simulink model "AMM_tracking"  (R2020a)
settings: Solver=VariableStepAuto  StartTime=0.0  StopTime=350  RelTol=1e-3
values from neighbouring files (symbols this model uses):
  a = (6371+h)*1e3    (= 6871000)    [AMM_main.m]    (also in Data.m)
  A_RW = sqrt([prop1;prop2;prop3]/(prop1+prop2+prop3))    [AMM_main.m]    (also in Data.m)
  A_t = [Ax;Ay;Az;Ax;Ay;Az;A_sp;A_sp;A_sp;A_sp;]    [AMM_main.m]    (also in Data.m)
  alpha = 0.005    [AMM_main.m]    (also in Data.m = 0.5)
  cd = 2.2    [AMM_main.m]    (also in Data.m)
  EH_dir = [0.152451072968615, 0.104990641908259, -0.112754568516865]    [AMM_main.m]
  EH_err = 0.25*pi/180    (= 0.00436332312999)    [AMM_main.m]
  Gyr_frq = 262    [AMM_main.m]
  init_DCM = DCM0_track    [AMM_main.m]    (also in Data.m = [0.097540404999410   0.957506835434298   0.970592781760616)
  init_gyro = w0_gyro_track    [AMM_main.m]
  init_hr = hr0_track    [AMM_main.m]
  init_orb = orb0_track    [AMM_main.m]    (also in Data.m = [e0,i0,O0,o0,th0])
  init_tumbl = w0_track    [AMM_main.m]    (also in Data.m = 10*pi/180*dir)
  Ir = 1e-7    (= 1e-07)    [AMM_main.m]    (also in Data.m)
  J = [Jx;Jy;Jz]    [AMM_main.m]    (also in Data.m)
  K1 = .05    (= 0.05)    [AMM_main.m]    (also in Data.m)
  K2 = 0.5*K1^2    (= 0.00125)    [AMM_main.m]    (also in Data.m)
  max_mx = 1.19    [AMM_main.m]    (also in Data.m)
  max_my = 1.19    [AMM_main.m]    (also in Data.m)
  MS_dir = [-0.144926348121151, 0.497003271606648, -0.275828501016873]    [AMM_main.m]
  MS_err = 2*pi/180    (= 0.0349065850399)    [AMM_main.m]
  MS_freq = 1    [AMM_main.m]    (also in Data.m)
  n = sqrt( mu / a^3 )    [AMM_main.m]    (also in Data.m)
  par_ind = [0.1;0.1;0.1]    [AMM_main.m]
  rho = [rho_sMB;rho_dMB;rho_sSP;rho_dSP]    [AMM_main.m]    (also in Data.m)
  rho_air = 4.39e-16 * 1e6/1e3    (= 4.39e-13)    [AMM_main.m]    (also in Data.m)
  RW_max_momentum = 400e-3    (= 0.4)    [AMM_main.m]    (also in Data.m)
  RW_max_torque = 100e-3    (= 0.1)    [AMM_main.m]    (also in Data.m)
  t0 = de_tumble.tout(end)    [AMM_main.m]
  wr = 100*pi/180    (= 1.74532925199)    [AMM_main.m]    (also in Data.m)
  ww_earth = 2*pi/(24*3600)*[0;0;1]    [AMM_main.m]    (also in Data.m)
libraries: dspmtrx3 x3, vrlib x3, simulink x3
(part 1 of 2)
settings Model: Creator=alejandrodemiguelmendiola  LastModifiedBy=alejandrodemiguelmendiola

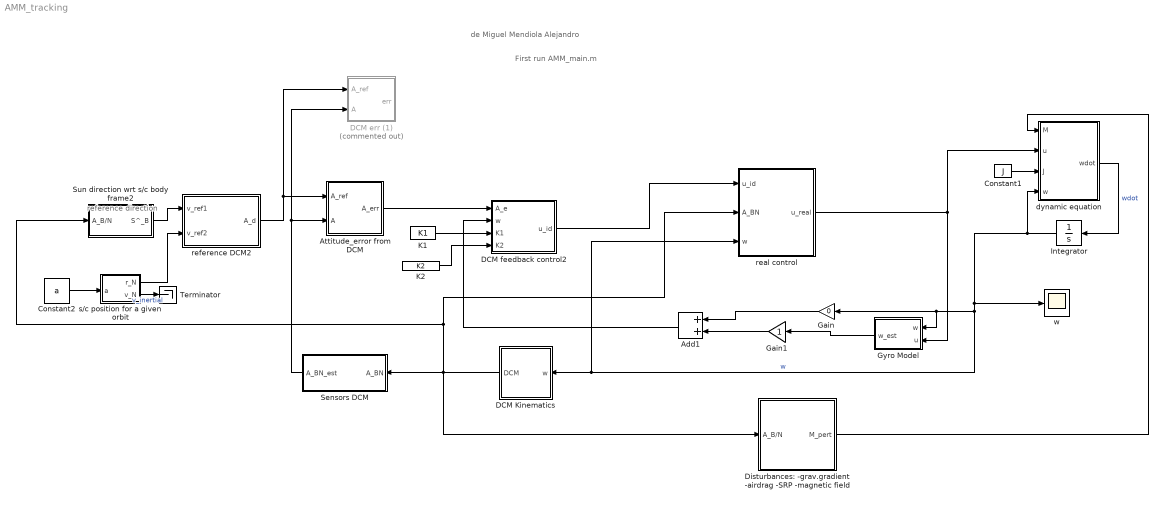
== system AMM_tracking ==
  note: reference direction
  note: First run AMM_main.m
  note: de Miguel Mendiola Alejandro
  Add1 : Sum
  Attitude_error from DCM : Subsystem
  Constant1 : Constant  Value=J
  Constant2 : Constant  Value=a
  DCM Kinematics : Subsystem
  DCM err (1) : Subsystem  Commented=on
  DCM feedback control2 : Subsystem
  Disturbances: -grav.gradient -airdrag -SRP -magnetic field : Subsystem
  Gain : Gain  Gain=0
  Gain1 : Gain
  Gyro Model : Subsystem
  Integrator : Integrator  InitialCondition=init_tumbl
  K1 : Constant  Value=K1
  K2 : Constant  Value=K2
  Sensors DCM : Subsystem
  Sun direction wrt s/c body frame2 : Subsystem
  Terminator : Terminator
  dynamic equation : MATLAB Function  TreatAsAtomicUnit=on
  "real control " : Subsystem
  reference DCM2 : Subsystem
  s/c position for a given orbit : Subsystem
  w : Scope
  wires:
  dynamic equation/1(wdot) -> Integrator/1  "wdot"
  Integrator/1 -> w/1, "real control "/3(w), DCM Kinematics/1(w), Gyro Model/1(w), Gain/1, dynamic equation/4(w)  "w"
  Disturbances: -grav.gradient -airdrag -SRP -magnetic field/1(M_pert) -> dynamic equation/1(M)
  Constant1/1 -> dynamic equation/3(J)
  Add1/1 -> DCM feedback control2/2(w)
  Gain1/1 -> Add1/2
  Gyro Model/1(w_est) -> Gain1/1
  Gain/1 -> Add1/1
  reference DCM2/1(A_d) -> DCM err (1)/1(A_ref), Attitude_error from DCM/1(A_ref)
  DCM Kinematics/1(DCM) -> "real control "/2(A_BN), Sun direction wrt s/c body frame2/1(A_B/N), Disturbances: -grav.gradient -airdrag -SRP -magnetic field/1(A_B/N), Sensors DCM/1(A_BN)
  Attitude_error from DCM/1(A_err) -> DCM feedback control2/1(A_e)
  Sensors DCM/1(A_BN_est) -> DCM err (1)/2(A), Attitude_error from DCM/2(A)
  K1/1 -> DCM feedback control2/3(K1)
  K2/1 -> DCM feedback control2/4(K2)
  Constant2/1 -> s/c position for a given orbit/1(a)
  s/c position for a given orbit/2(v_N) -> Terminator/1  "v_inertial"
  s/c position for a given orbit/1(r_N) -> reference DCM2/2(v_ref2)
  Sun direction wrt s/c body frame2/1(S^_B) -> reference DCM2/1(v_ref1)
  "real control "/1(u_real) -> dynamic equation/2(u), Gyro Model/2(u)
  DCM feedback control2/1(u_id) -> "real control "/1(u_id)

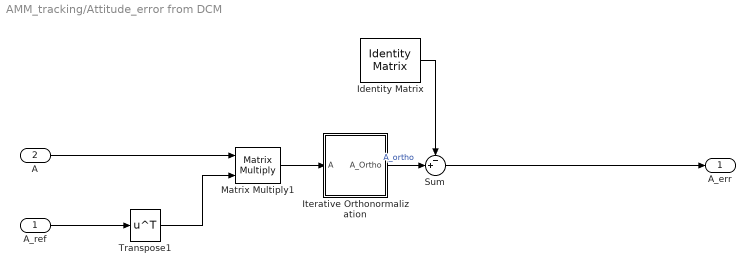
== system AMM_tracking/Attitude_error from DCM ==
  A_ref : Inport
  A : Inport  Port=2
  Identity Matrix : dspmtrx3/Identity Matrix  Inherit=off  N=3  Ts=1  dataType=double  isSigned=on  wordLen=16  udDataType=sfix(16)  fracBitsMode=Best precision  numFracBits=15  OutDataTypeStr=double  LastOutDataTypeStr=double
  Iterative Orthonormalization : Subsystem
  Matrix Multiply1 : Product  Multiplication=Matrix(*)
  Sum : Sum  Inputs=-+|
  Transpose1 : Math  Operator=transpose  SaturateOnIntegerOverflow=on
  A_err : Outport
  wires:
  A_ref/1 -> Transpose1/1
  Transpose1/1 -> Matrix Multiply1/2
  A/1 -> Matrix Multiply1/1
  Sum/1 -> A_err/1
  Identity Matrix/1 -> Sum/1
  Matrix Multiply1/1 -> Iterative Orthonormalization/1(A)
  Iterative Orthonormalization/1(A_Ortho) -> Sum/2  "A_ortho"

== system AMM_tracking/DCM Kinematics ==
  w : Inport
  Integrator : Integrator  InitialCondition=init_DCM
  Iterative Orthonormalization : Subsystem
  Product1 : Product  Multiplication=Matrix(*)
  Unary Minus : UnaryMinus
  hat : MATLAB Function  TreatAsAtomicUnit=on
  DCM : Outport
  wires:
  Unary Minus/1 -> Integrator/1  "Adot"
  hat/1(w_hat) -> Product1/1
  Product1/1 -> Unary Minus/1
  w/1 -> hat/1(w)
  Iterative Orthonormalization/1(A_Ortho) -> Product1/2, DCM/1  "A_ortho"
  Integrator/1 -> Iterative Orthonormalization/1(A)  "A"

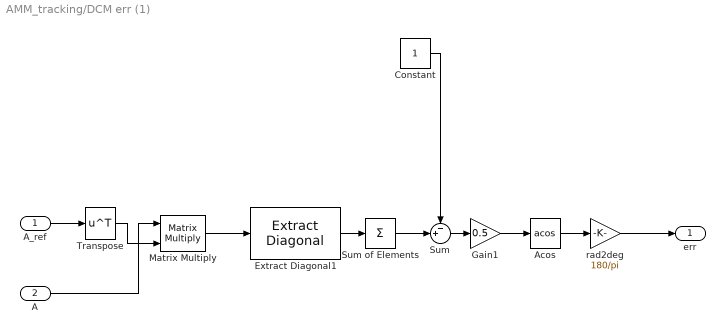
== system AMM_tracking/DCM err (1) ==
  A_ref : Inport
  A : Inport  Port=2
  Acos : Trigonometry  Operator=acos
  Constant : Constant
  Extract Diagonal1 : dspmtrx3/Extract Diagonal
      settings: SourceProductBaseCode=DS
  Gain1 : Gain  Gain=0.5
  Matrix Multiply : Product  Multiplication=Matrix(*)
  Sum : Sum  Inputs=-+|
  Sum of Elements : Sum  Inputs=+
  Transpose : Math  Operator=transpose  SaturateOnIntegerOverflow=on
  rad2deg : Gain  Gain=180/pi
  err : Outport
  wires:
  Matrix Multiply/1 -> Extract Diagonal1/1
  Extract Diagonal1/1 -> Sum of Elements/1
  A_ref/1 -> Transpose/1
  Sum/1 -> Gain1/1
  Acos/1 -> rad2deg/1
  Sum of Elements/1 -> Sum/2
  Constant/1 -> Sum/1
  rad2deg/1 -> err/1
  Gain1/1 -> Acos/1
  A/1 -> Matrix Multiply/1
  Transpose/1 -> Matrix Multiply/2

== system AMM_tracking/DCM feedback control2 ==
  A_e : Inport
  w : Inport  Port=2
  K1 : Inport  Port=3
  K2 : Inport  Port=4
  Constant2 : Constant  Value=J
  DCM feedback : MATLAB Function  TreatAsAtomicUnit=on
  u_id : Outport
  wires:
  DCM feedback/1(u) -> u_id/1
  A_e/1 -> DCM feedback/2(A_e)
  Constant2/1 -> DCM feedback/5(J)
  K2/1 -> DCM feedback/4(K2)
  w/1 -> DCM feedback/1(w)
  K1/1 -> DCM feedback/3(K1)

== system AMM_tracking/Disturbances: -grav.gradient -airdrag -SRP -magnetic field ==
  A_B/N : Inport
  Add : Sum  Inputs=++++
  SRP moment : Subsystem
  air drag : Subsystem
  gravity gradient : Subsystem
  magnetic torque : Subsystem
  M_pert : Outport
  wires:
  magnetic torque/1(magnetic torque M) -> Add/1
  SRP moment/1(T_srp) -> Add/2
  gravity gradient/1(G) -> Add/4
  Add/1 -> M_pert/1
  air drag/1(M_drag) -> Add/3
  A_B/N/1 -> magnetic torque/1(A_BN), SRP moment/1(A_B/N), gravity gradient/1(A_BN), air drag/1(A_B/N)

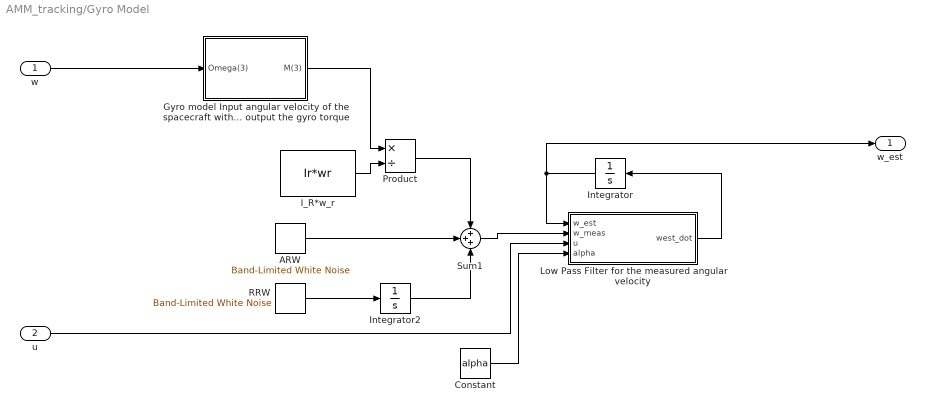
== system AMM_tracking/Gyro Model ==
  w : Inport
  u : Inport  Port=2
  ARW : simulink/Sources/Band-Limited White Noise  Cov=Gyr_ARW  Ts=1/Gyr_frq  seed=[23341]
  Constant : Constant  Value=alpha
  Gyro model Input angular velocity of the spacecraft with output the gyro torque : Subsystem
  I_R*w_r : Constant  Value=Ir*wr
  Integrator : Integrator  InitialCondition=init_gyro
  Integrator2 : Integrator  InitialCondition=pi/180/3600*[1,1,1]'
  Low Pass Filter for the measured angular velocity : MATLAB Function  TreatAsAtomicUnit=on
  Product : Product  Inputs=*/
  RRW : simulink/Sources/Band-Limited White Noise  Cov=Gyr_RRW  Ts=1/Gyr_frq  seed=[23341]
  Sum1 : Sum  Inputs=+++
  w_est : Outport
  wires:
  Gyro model Input angular velocity of the spacecraft with output the gyro torque/1(M(3)) -> Product/1
  Low Pass Filter for the measured angular velocity/1(west_dot) -> Integrator/1
  I_R*w_r/1 -> Product/2
  Integrator/1 -> w_est/1, Low Pass Filter for the measured angular velocity/1(w_est)
  Sum1/1 -> Low Pass Filter for the measured angular velocity/2(w_meas)
  w/1 -> Gyro model Input angular velocity of the spacecraft with output the gyro torque/1(Omega(3))
  u/1 -> Low Pass Filter for the measured angular velocity/3(u)
  Integrator2/1 -> Sum1/3
  Product/1 -> Sum1/1
  RRW/1 -> Integrator2/1
  ARW/1 -> Sum1/2
  Constant/1 -> Low Pass Filter for the measured angular velocity/4(alpha)

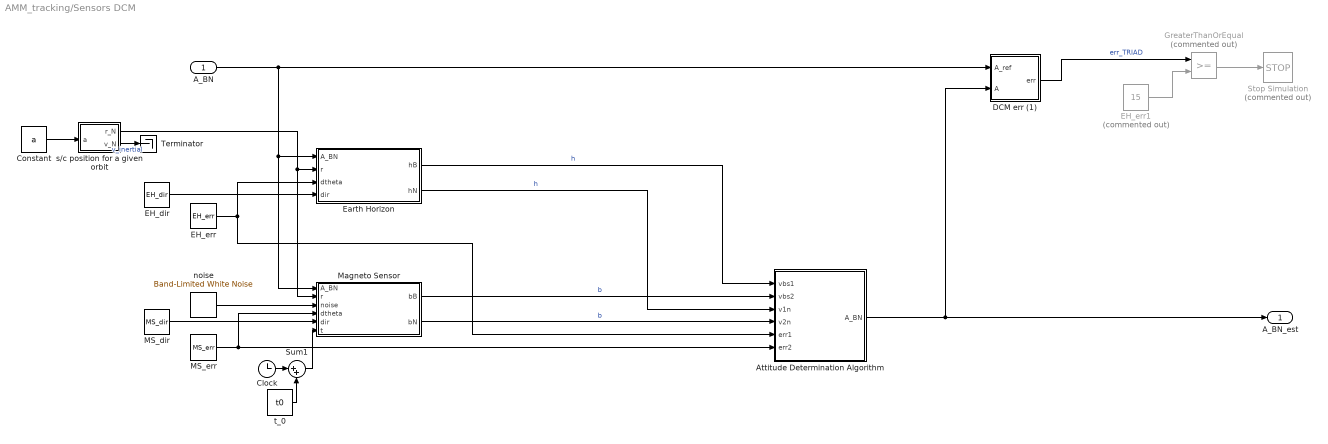
== system AMM_tracking/Sensors DCM ==
  A_BN : Inport
  Attitude Determination Algorithm : MATLAB Function  TreatAsAtomicUnit=on
  Clock : Clock
  Constant : Constant  Value=a
  DCM err (1) : Subsystem
  EH_dir : Constant  Value=EH_dir
  EH_err : Constant  Value=EH_err
  EH_err1 : Constant  Commented=on  Value=15
  Earth Horizon : MATLAB Function  TreatAsAtomicUnit=on
  GreaterThanOrEqual : RelationalOperator  Commented=on  OutDataTypeStr=boolean  RndMeth=Simplest
  MS_dir : Constant  Value=MS_dir
  MS_err : Constant  Value=MS_err
  Magneto Sensor : MATLAB Function  TreatAsAtomicUnit=on
  Stop Simulation : Stop  Commented=on
  Sum1 : Sum  Inputs=|++
  Terminator : Terminator
  noise : simulink/Sources/Band-Limited White Noise  Cov=MS_noise  Ts=MS_freq  seed=[23341]
  s/c position for a given orbit : Subsystem
  t_0 : Constant  Value=t0
  A_BN_est : Outport
  wires:
  s/c position for a given orbit/1(r_N) -> Earth Horizon/2(r), Magneto Sensor/2(r)
  EH_err/1 -> Earth Horizon/3(dtheta), Attitude Determination Algorithm/5(err1)
  Earth Horizon/1(hB) -> Attitude Determination Algorithm/1(vbs1)  "h"
  MS_err/1 -> Magneto Sensor/4(dtheta), Attitude Determination Algorithm/6(err2)
  Magneto Sensor/1(bB) -> Attitude Determination Algorithm/2(vbs2)  "b"
  Clock/1 -> Sum1/1
  A_BN/1 -> DCM err (1)/1(A_ref), Magneto Sensor/1(A_BN), Earth Horizon/1(A_BN)
  DCM err (1)/1(err) -> GreaterThanOrEqual/1  "err_TRIAD"
  Attitude Determination Algorithm/1(A_BN) -> A_BN_est/1, DCM err (1)/2(A)
  Sum1/1 -> Magneto Sensor/6(t)
  noise/1 -> Magneto Sensor/3(noise)
  MS_dir/1 -> Magneto Sensor/5(dir)
  EH_dir/1 -> Earth Horizon/4(dir)
  t_0/1 -> Sum1/2
  Earth Horizon/2(hN) -> Attitude Determination Algorithm/3(v1n)  "h"
  Magneto Sensor/2(bN) -> Attitude Determination Algorithm/4(v2n)  "b"
  GreaterThanOrEqual/1 -> Stop Simulation/1
  EH_err1/1 -> GreaterThanOrEqual/2
  Constant/1 -> s/c position for a given orbit/1(a)
  s/c position for a given orbit/2(v_N) -> Terminator/1  "v_inertial"

== system AMM_tracking/Sun direction wrt s//c body frame2 ==
  A_B/N : Inport
  Add : Sum
  Clock : Clock
  Constant1 : Constant  Value=t0
  Product3 : Product  Multiplication=Matrix(*)
  Sun's direction : MATLAB Function  TreatAsAtomicUnit=on
  S^_B : Outport
  wires:
  Product3/1 -> S^_B/1
  A_B/N/1 -> Product3/1
  Sun's direction/1(S_N) -> Product3/2  "S^_N"
  Clock/1 -> Add/1
  Add/1 -> Sun's direction/1(t)
  Constant1/1 -> Add/2

== system AMM_tracking/real control  ==
  u_id : Inport
  A_BN : Inport  Port=2
  w : Inport  Port=3
  Add : Sum
  MT+RW control1 : Subsystem  Commented=on
  RW : Subsystem
  u_real : Outport
  wires:
  RW/1(u_r) -> Add/1  "u_real 4RW"
  w/1 -> RW/2(w), MT+RW control1/1(w)
  A_BN/1 -> MT+RW control1/3(A_BN)
  Add/1 -> u_real/1
  MT+RW control1/1(u_real) -> Add/2
  u_id/1 -> RW/1(u_id), MT+RW control1/2(M_c)

== system AMM_tracking/reference DCM2 ==
  v_ref1 : Inport
  v_ref2 : Inport  Port=2
  DCM_ref : MATLAB Function  TreatAsAtomicUnit=on
  A_d : Outport
  wires:
  DCM_ref/1(A_d) -> A_d/1
  v_ref1/1 -> DCM_ref/1(v_ref)
  v_ref2/1 -> DCM_ref/2(r_sc)

== system AMM_tracking/s//c position for a given orbit ==
  a : Inport
  Earth's position : MATLAB Function  TreatAsAtomicUnit=on
  orb_elements dynamics : Subsystem
  r_N : Outport
  v_N : Outport  Port=2
  wires:
  Earth's position/1(r_N) -> r_N/1  "r_N"
  orb_elements dynamics/1(orb_elements) -> Earth's position/2(orb_elements)
  a/1 -> orb_elements dynamics/1(a), Earth's position/1(a)  "a"
  Earth's position/2(v_N) -> v_N/1

== system AMM_tracking/Attitude_error from DCM/Iterative Orthonormalization ==
  note: Uncomment if needed
      | With 2 blocks working:
      | Error ~1e-16 up to t=1e6
      | Error ~1e-14 up to t=1e7
  A : Inport
  Ortho DCM : Subsystem
  Ortho DCM1 : Subsystem
  Ortho DCM2 : Subsystem
  Ortho DCM3 : Subsystem  Commented=through
  Ortho DCM4 : Subsystem  Commented=through
  A_Ortho : Outport
  wires:
  Ortho DCM1/1(A_ortho) -> Ortho DCM2/1(A)
  Ortho DCM/1(A_ortho) -> Ortho DCM1/1(A)
  Ortho DCM3/1(A_ortho) -> Ortho DCM4/1(A)
  Ortho DCM2/1(A_ortho) -> Ortho DCM3/1(A)
  A/1 -> Ortho DCM/1(A)
  Ortho DCM4/1(A_ortho) -> A_Ortho/1

== system AMM_tracking/DCM Kinematics/Iterative Orthonormalization ==
  note: Uncomment if needed
      | With 2 blocks working:
      | Error ~1e-16 up to t=1e6
      | Error ~1e-14 up to t=1e7
  A : Inport
  Ortho DCM : Subsystem
  Ortho DCM1 : Subsystem
  Ortho DCM2 : Subsystem  Commented=through
  Ortho DCM3 : Subsystem  Commented=through
  Ortho DCM4 : Subsystem  Commented=through
  A_Ortho : Outport
  wires:
  Ortho DCM1/1(A_ortho) -> Ortho DCM2/1(A)
  Ortho DCM/1(A_ortho) -> Ortho DCM1/1(A)
  Ortho DCM3/1(A_ortho) -> Ortho DCM4/1(A)
  Ortho DCM2/1(A_ortho) -> Ortho DCM3/1(A)
  A/1 -> Ortho DCM/1(A)
  Ortho DCM4/1(A_ortho) -> A_Ortho/1

== system AMM_tracking/Disturbances: -grav.gradient -airdrag -SRP -magnetic field/SRP moment ==
  A_B/N : Inport
  Area : Constant  Value=A_t
  SRP disturbance torque : MATLAB Function  TreatAsAtomicUnit=on
  Sun direction wrt s/c body frame : Subsystem
  optical properties : Constant  Value=rho
  T_srp : Outport
  wires:
  A_B/N/1 -> Sun direction wrt s/c body frame/1(A_B/N)
  SRP disturbance torque/1(T_srp) -> T_srp/1
  Sun direction wrt s/c body frame/1(S^_B) -> SRP disturbance torque/1(S_B)
  Area/1 -> SRP disturbance torque/2(A)
  optical properties/1 -> SRP disturbance torque/3(rho)

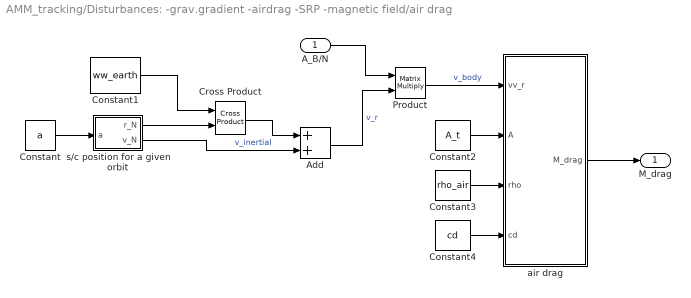
== system AMM_tracking/Disturbances: -grav.gradient -airdrag -SRP -magnetic field/air drag ==
  A_B/N : Inport
  Add : Sum
  Constant : Constant  Value=a
  Constant1 : Constant  Value=ww_earth
  Constant2 : Constant  Value=A_t
  Constant3 : Constant  Value=rho_air
  Constant4 : Constant  Value=cd
  Cross Product : vrlib/Utilities/Cross Product
  Product : Product  Multiplication=Matrix(*)
  air drag : MATLAB Function  TreatAsAtomicUnit=on
  s/c position for a given orbit : Subsystem
  M_drag : Outport
  wires:
  air drag/1(M_drag) -> M_drag/1
  A_B/N/1 -> Product/1
  Product/1 -> air drag/1(vv_r)  "v_body"
  Constant/1 -> s/c position for a given orbit/1(a)
  s/c position for a given orbit/1(r_N) -> Cross Product/2
  Constant1/1 -> Cross Product/1
  Cross Product/1 -> Add/1
  s/c position for a given orbit/2(v_N) -> Add/2  "v_inertial"
  Add/1 -> Product/2  "v_r"
  Constant2/1 -> air drag/2(A)
  Constant4/1 -> air drag/4(cd)
  Constant3/1 -> air drag/3(rho)

== system AMM_tracking/Disturbances: -grav.gradient -airdrag -SRP -magnetic field/gravity gradient ==
  A_BN : Inport
  A_N/L : Subsystem
  Product : Product  Multiplication=Matrix(*)
  gravity gradient : MATLAB Function  TreatAsAtomicUnit=on
  mean motion : Constant  Value=n
  moment of inertia : Constant  Value=J
  G : Outport
  wires:
  gravity gradient/1(G) -> G/1
  A_N/L/1(A_N/L) -> Product/2
  A_BN/1 -> Product/1
  Product/1 -> gravity gradient/1(A_BL)
  moment of inertia/1 -> gravity gradient/2(J)
  mean motion/1 -> gravity gradient/3(n)

== system AMM_tracking/Disturbances: -grav.gradient -airdrag -SRP -magnetic field/magnetic torque ==
  A_BN : Inport
  Cross Product : vrlib/Utilities/Cross Product
  m (worst case scenario) : Constant  Value=par_ind
  magnetic model : Subsystem
  magnetic torque M : Outport
  wires:
  magnetic model/1(b_B) -> Cross Product/2  "b_B"
  m (worst case scenario)/1 -> Cross Product/1
  Cross Product/1 -> magnetic torque M/1  "M"
  A_BN/1 -> magnetic model/1(A_BN)

== system AMM_tracking/Gyro Model/Gyro model Input angular velocity of the spacecraft with output the gyro torque ==
  Omega(3) : Inport
  Integrator2 : Integrator  InitialCondition=[0;0;0;0;0;0]
  MATLAB Function1 : MATLAB Function  TreatAsAtomicUnit=on
  M(3) : Outport
  wires:
  Integrator2/1 -> MATLAB Function1/1(x)
  MATLAB Function1/1(x_dot) -> Integrator2/1
  Omega(3)/1 -> MATLAB Function1/2(om)
  MATLAB Function1/2(M) -> M(3)/1

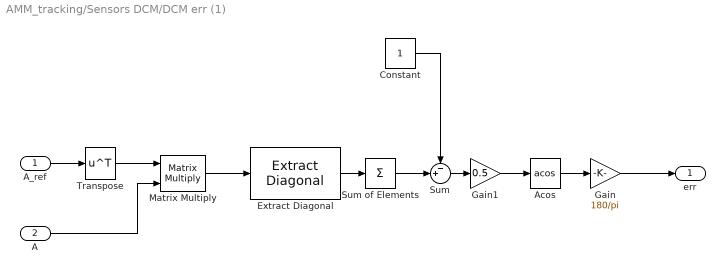
== system AMM_tracking/Sensors DCM/DCM err (1) ==
  A_ref : Inport
  A : Inport  Port=2
  Acos : Trigonometry  Operator=acos
  Constant : Constant
  Extract Diagonal : dspmtrx3/Extract Diagonal
      settings: SourceProductBaseCode=DS
  Gain : Gain  Gain=180/pi
  Gain1 : Gain  Gain=0.5
  Matrix Multiply : Product  Multiplication=Matrix(*)
  Sum : Sum  Inputs=-+|
  Sum of Elements : Sum  Inputs=+
  Transpose : Math  Operator=transpose  SaturateOnIntegerOverflow=on
  err : Outport
  wires:
  Transpose/1 -> Matrix Multiply/1
  Matrix Multiply/1 -> Extract Diagonal/1
  Extract Diagonal/1 -> Sum of Elements/1
  A/1 -> Matrix Multiply/2
  A_ref/1 -> Transpose/1
  Sum/1 -> Gain1/1
  Acos/1 -> Gain/1
  Sum of Elements/1 -> Sum/2
  Constant/1 -> Sum/1
  Gain/1 -> err/1
  Gain1/1 -> Acos/1

== system AMM_tracking/Sensors DCM/s//c position for a given orbit ==
  a : Inport
  Earth's position : MATLAB Function  TreatAsAtomicUnit=on
  orb_elements dynamics : Subsystem
  r_N : Outport
  v_N : Outport  Port=2
  wires:
  Earth's position/1(r_N) -> r_N/1  "r_N"
  orb_elements dynamics/1(orb_elements) -> Earth's position/2(orb_elements)
  a/1 -> orb_elements dynamics/1(a), Earth's position/1(a)  "a"
  Earth's position/2(v_N) -> v_N/1

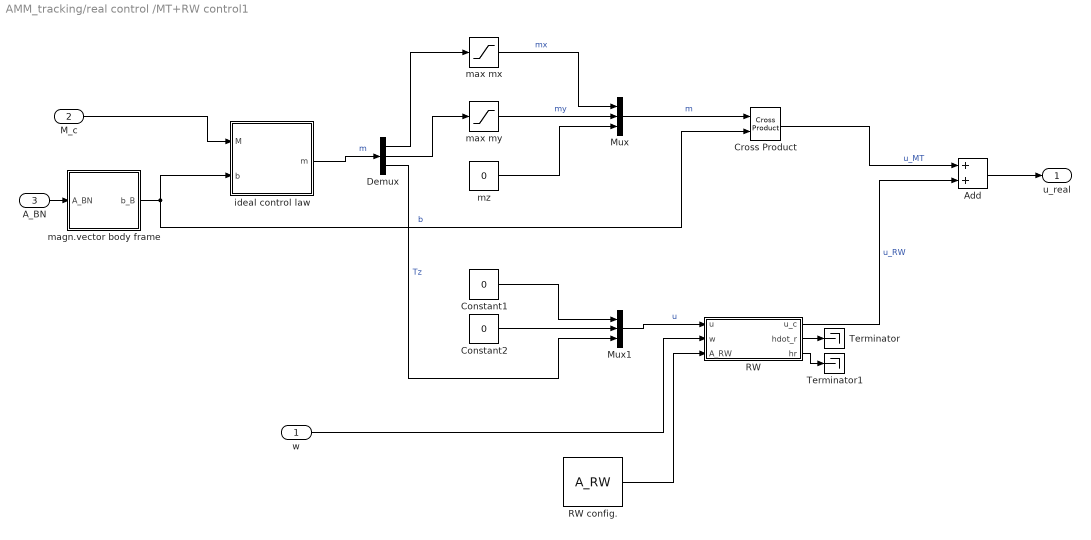
== system AMM_tracking/real control /MT+RW control1 ==
  w : Inport
  M_c : Inport  Port=2
  A_BN : Inport  Port=3
  " RW" : Subsystem
  Add : Sum
  Constant1 : Constant  Value=0
  Constant2 : Constant  Value=0
  Cross Product : vrlib/Utilities/Cross Product
  Demux : Demux  Outputs=3
  Mux : Mux  Inputs=3
  Mux1 : Mux  Inputs=3
  RW config. : Constant  Value=A_RW
  Terminator : Terminator
  Terminator1 : Terminator
  ideal control law : MATLAB Function  TreatAsAtomicUnit=on
  magn.vector body frame : Subsystem
  max mx : Saturate  UpperLimit=max_mx  LowerLimit=-max_mx
  max my : Saturate  UpperLimit=max_my  LowerLimit=-max_my
  mz : Constant  Value=0
  u_real : Outport
  wires:
  magn.vector body frame/1(b_B) -> Cross Product/2, ideal control law/2(b)  "b"
  M_c/1 -> ideal control law/1(M)
  A_BN/1 -> magn.vector body frame/1(A_BN)
  ideal control law/1(m) -> Demux/1  "m"
  Mux/1 -> Cross Product/1  "m"
  max mx/1 -> Mux/1  "mx"
  Demux/2 -> max my/1
  Demux/1 -> max mx/1
  max my/1 -> Mux/2  "my"
  mz/1 -> Mux/3
  Constant2/1 -> Mux1/2
  Demux/3 -> Mux1/3  "Tz"
  Constant1/1 -> Mux1/1
  Mux1/1 -> " RW"/1(u)  "u"
  Cross Product/1 -> Add/1  "u_MT"
  w/1 -> " RW"/2(w)
  RW config./1 -> " RW"/3(A_RW)
  " RW"/1(u_c) -> Add/2  "u_RW"
  Add/1 -> u_real/1
  " RW"/2(hdot_r) -> Terminator/1
  " RW"/3(hr) -> Terminator1/1

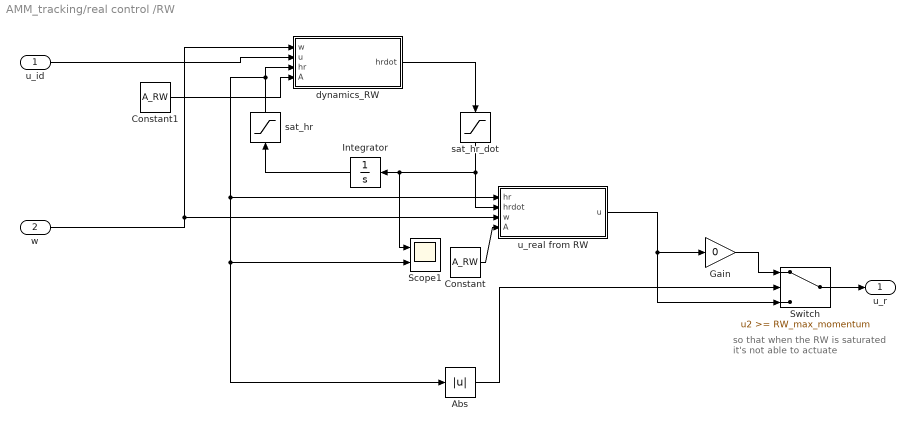
== system AMM_tracking/real control /RW ==
  note: so that when the RW is saturated
      | it's not able to actuate
  u_id : Inport
  w : Inport  Port=2
  Abs : Abs
  Constant : Constant  Value=A_RW
  Constant1 : Constant  Value=A_RW
  Gain : Gain  Gain=0
  Integrator : Integrator  InitialCondition=init_hr
  Scope1 : Scope  NumInputPorts=2
  Switch : Switch  Threshold=RW_max_momentum
  dynamics_RW : MATLAB Function  TreatAsAtomicUnit=on
  sat_hr : Saturate  UpperLimit=RW_max_momentum  LowerLimit=-RW_max_momentum
  sat_hr_dot : Saturate  UpperLimit=RW_max_torque  LowerLimit=-RW_max_torque
  u_real from RW : MATLAB Function  TreatAsAtomicUnit=on
  u_r : Outport
  wires:
  w/1 -> dynamics_RW/1(w), u_real from RW/3(w)
  u_id/1 -> dynamics_RW/2(u)
  dynamics_RW/1(hrdot) -> sat_hr_dot/1
  Integrator/1 -> sat_hr/1
  sat_hr/1 -> dynamics_RW/3(hr), Abs/1, Scope1/2, u_real from RW/1(hr)
  sat_hr_dot/1 -> Scope1/1, Integrator/1, u_real from RW/2(hrdot)
  Constant/1 -> u_real from RW/4(A)
  Constant1/1 -> dynamics_RW/4(A)
  Switch/1 -> u_r/1
  Abs/1 -> Switch/2
  u_real from RW/1(u) -> Gain/1, Switch/3
  Gain/1 -> Switch/1

== system AMM_tracking/s//c position for a given orbit/orb_elements dynamics ==
  a : Inport
  Integrator : Integrator  InitialCondition=init_orb
  sat motion : MATLAB Function  TreatAsAtomicUnit=on
  orb_elements : Outport
  wires:
  Integrator/1 -> sat motion/2(orb_elements), orb_elements/1  "orb_elements"
  sat motion/1(orb_elements_dot) -> Integrator/1
  a/1 -> sat motion/1(a)

== system AMM_tracking/Attitude_error from DCM/Iterative Orthonormalization/Ortho DCM ==
  A : Inport
  Gain : Gain  Gain=1.5
  Gain1 : Gain  Gain=0.5
  Matrix Multiply : Product  Multiplication=Matrix(*)
  Matrix Multiply1 : Product  Multiplication=Matrix(*)
  Sum : Sum  Inputs=|+-
  Transpose : Math  Operator=transpose  SaturateOnIntegerOverflow=on
  A_ortho : Outport
  wires:
  Sum/1 -> A_ortho/1
  Gain/1 -> Sum/1
  A/1 -> Matrix Multiply1/2, Transpose/1, Matrix Multiply/1, Gain/1
  Gain1/1 -> Sum/2
  Transpose/1 -> Matrix Multiply/2
  Matrix Multiply/1 -> Matrix Multiply1/1
  Matrix Multiply1/1 -> Gain1/1

== system AMM_tracking/Attitude_error from DCM/Iterative Orthonormalization/Ortho DCM1 ==
  A : Inport
  Gain : Gain  Gain=1.5
  Gain1 : Gain  Gain=0.5
  Matrix Multiply : Product  Multiplication=Matrix(*)
  Matrix Multiply1 : Product  Multiplication=Matrix(*)
  Sum : Sum  Inputs=|+-
  Transpose : Math  Operator=transpose  SaturateOnIntegerOverflow=on
  A_ortho : Outport
  wires:
  Sum/1 -> A_ortho/1
  Gain/1 -> Sum/1
  A/1 -> Matrix Multiply1/2, Transpose/1, Matrix Multiply/1, Gain/1
  Gain1/1 -> Sum/2
  Transpose/1 -> Matrix Multiply/2
  Matrix Multiply/1 -> Matrix Multiply1/1
  Matrix Multiply1/1 -> Gain1/1

== system AMM_tracking/Attitude_error from DCM/Iterative Orthonormalization/Ortho DCM2 ==
  A : Inport
  Gain : Gain  Gain=1.5
  Gain1 : Gain  Gain=0.5
  Matrix Multiply : Product  Multiplication=Matrix(*)
  Matrix Multiply1 : Product  Multiplication=Matrix(*)
  Sum : Sum  Inputs=|+-
  Transpose : Math  Operator=transpose  SaturateOnIntegerOverflow=on
  A_ortho : Outport
  wires:
  Sum/1 -> A_ortho/1
  Gain/1 -> Sum/1
  A/1 -> Matrix Multiply1/2, Transpose/1, Matrix Multiply/1, Gain/1
  Gain1/1 -> Sum/2
  Transpose/1 -> Matrix Multiply/2
  Matrix Multiply/1 -> Matrix Multiply1/1
  Matrix Multiply1/1 -> Gain1/1

== system AMM_tracking/Attitude_error from DCM/Iterative Orthonormalization/Ortho DCM3 ==
  A : Inport
  Gain : Gain  Gain=1.5
  Gain1 : Gain  Gain=0.5
  Matrix Multiply : Product  Multiplication=Matrix(*)
  Matrix Multiply1 : Product  Multiplication=Matrix(*)
  Sum : Sum  Inputs=|+-
  Transpose : Math  Operator=transpose  SaturateOnIntegerOverflow=on
  A_ortho : Outport
  wires:
  Sum/1 -> A_ortho/1
  Gain/1 -> Sum/1
  A/1 -> Matrix Multiply1/2, Transpose/1, Matrix Multiply/1, Gain/1
  Gain1/1 -> Sum/2
  Transpose/1 -> Matrix Multiply/2
  Matrix Multiply/1 -> Matrix Multiply1/1
  Matrix Multiply1/1 -> Gain1/1

== system AMM_tracking/Attitude_error from DCM/Iterative Orthonormalization/Ortho DCM4 ==
  A : Inport
  Gain : Gain  Gain=1.5
  Gain1 : Gain  Gain=0.5
  Matrix Multiply : Product  Multiplication=Matrix(*)
  Matrix Multiply1 : Product  Multiplication=Matrix(*)
  Sum : Sum  Inputs=|+-
  Transpose : Math  Operator=transpose  SaturateOnIntegerOverflow=on
  A_ortho : Outport
  wires:
  Sum/1 -> A_ortho/1
  Gain/1 -> Sum/1
  A/1 -> Matrix Multiply1/2, Transpose/1, Matrix Multiply/1, Gain/1
  Gain1/1 -> Sum/2
  Transpose/1 -> Matrix Multiply/2
  Matrix Multiply/1 -> Matrix Multiply1/1
  Matrix Multiply1/1 -> Gain1/1

== system AMM_tracking/DCM Kinematics/Iterative Orthonormalization/Ortho DCM ==
  A : Inport
  Gain : Gain  Gain=1.5
  Gain1 : Gain  Gain=0.5
  Matrix Multiply : Product  Multiplication=Matrix(*)
  Matrix Multiply1 : Product  Multiplication=Matrix(*)
  Sum : Sum  Inputs=|+-
  Transpose : Math  Operator=transpose  SaturateOnIntegerOverflow=on
  A_ortho : Outport
  wires:
  Sum/1 -> A_ortho/1
  Gain/1 -> Sum/1
  A/1 -> Matrix Multiply1/2, Transpose/1, Matrix Multiply/1, Gain/1
  Gain1/1 -> Sum/2
  Transpose/1 -> Matrix Multiply/2
  Matrix Multiply/1 -> Matrix Multiply1/1
  Matrix Multiply1/1 -> Gain1/1

== system AMM_tracking/DCM Kinematics/Iterative Orthonormalization/Ortho DCM1 ==
  A : Inport
  Gain : Gain  Gain=1.5
  Gain1 : Gain  Gain=0.5
  Matrix Multiply : Product  Multiplication=Matrix(*)
  Matrix Multiply1 : Product  Multiplication=Matrix(*)
  Sum : Sum  Inputs=|+-
  Transpose : Math  Operator=transpose  SaturateOnIntegerOverflow=on
  A_ortho : Outport
  wires:
  Sum/1 -> A_ortho/1
  Gain/1 -> Sum/1
  A/1 -> Matrix Multiply1/2, Transpose/1, Matrix Multiply/1, Gain/1
  Gain1/1 -> Sum/2
  Transpose/1 -> Matrix Multiply/2
  Matrix Multiply/1 -> Matrix Multiply1/1
  Matrix Multiply1/1 -> Gain1/1

== system AMM_tracking/DCM Kinematics/Iterative Orthonormalization/Ortho DCM2 ==
  A : Inport
  Gain : Gain  Gain=1.5
  Gain1 : Gain  Gain=0.5
  Matrix Multiply : Product  Multiplication=Matrix(*)
  Matrix Multiply1 : Product  Multiplication=Matrix(*)
  Sum : Sum  Inputs=|+-
  Transpose : Math  Operator=transpose  SaturateOnIntegerOverflow=on
  A_ortho : Outport
  wires:
  Sum/1 -> A_ortho/1
  Gain/1 -> Sum/1
  A/1 -> Matrix Multiply1/2, Transpose/1, Matrix Multiply/1, Gain/1
  Gain1/1 -> Sum/2
  Transpose/1 -> Matrix Multiply/2
  Matrix Multiply/1 -> Matrix Multiply1/1
  Matrix Multiply1/1 -> Gain1/1

== system AMM_tracking/DCM Kinematics/Iterative Orthonormalization/Ortho DCM3 ==
  A : Inport
  Gain : Gain  Gain=1.5
  Gain1 : Gain  Gain=0.5
  Matrix Multiply : Product  Multiplication=Matrix(*)
  Matrix Multiply1 : Product  Multiplication=Matrix(*)
  Sum : Sum  Inputs=|+-
  Transpose : Math  Operator=transpose  SaturateOnIntegerOverflow=on
  A_ortho : Outport
  wires:
  Sum/1 -> A_ortho/1
  Gain/1 -> Sum/1
  A/1 -> Matrix Multiply1/2, Transpose/1, Matrix Multiply/1, Gain/1
  Gain1/1 -> Sum/2
  Transpose/1 -> Matrix Multiply/2
  Matrix Multiply/1 -> Matrix Multiply1/1
  Matrix Multiply1/1 -> Gain1/1

== system AMM_tracking/DCM Kinematics/Iterative Orthonormalization/Ortho DCM4 ==
  A : Inport
  Gain : Gain  Gain=1.5
  Gain1 : Gain  Gain=0.5
  Matrix Multiply : Product  Multiplication=Matrix(*)
  Matrix Multiply1 : Product  Multiplication=Matrix(*)
  Sum : Sum  Inputs=|+-
  Transpose : Math  Operator=transpose  SaturateOnIntegerOverflow=on
  A_ortho : Outport
  wires:
  Sum/1 -> A_ortho/1
  Gain/1 -> Sum/1
  A/1 -> Matrix Multiply1/2, Transpose/1, Matrix Multiply/1, Gain/1
  Gain1/1 -> Sum/2
  Transpose/1 -> Matrix Multiply/2
  Matrix Multiply/1 -> Matrix Multiply1/1
  Matrix Multiply1/1 -> Gain1/1

== system AMM_tracking/Disturbances: -grav.gradient -airdrag -SRP -magnetic field/SRP moment/Sun direction wrt s//c body frame ==
  A_B/N : Inport
  Add : Sum
  Clock : Clock
  Constant1 : Constant  Value=t0
  Product3 : Product  Multiplication=Matrix(*)
  Sun's direction : MATLAB Function  TreatAsAtomicUnit=on
  S^_B : Outport
  wires:
  Product3/1 -> S^_B/1
  A_B/N/1 -> Product3/1
  Sun's direction/1(S_N) -> Product3/2  "S^_N"
  Clock/1 -> Add/1
  Add/1 -> Sun's direction/1(t)
  Constant1/1 -> Add/2

== system AMM_tracking/Disturbances: -grav.gradient -airdrag -SRP -magnetic field/air drag/s//c position for a given orbit ==
  a : Inport
  Earth's position : MATLAB Function  TreatAsAtomicUnit=on
  orb_elements dynamics : Subsystem
  r_N : Outport
  v_N : Outport  Port=2
  wires:
  Earth's position/1(r_N) -> r_N/1  "r_N"
  orb_elements dynamics/1(orb_elements) -> Earth's position/2(orb_elements)
  a/1 -> orb_elements dynamics/1(a), Earth's position/1(a)  "a"
  Earth's position/2(v_N) -> v_N/1

== system AMM_tracking/Disturbances: -grav.gradient -airdrag -SRP -magnetic field/gravity gradient/A_N//L ==
  Add : Sum
  Clock : Clock
  Constant1 : Constant  Value=t0
  MATLAB Function1 : MATLAB Function  TreatAsAtomicUnit=on
  Transpose : Math  Operator=transpose  SaturateOnIntegerOverflow=on
  mean motion : Constant  Value=n
  A_N/L : Outport
  wires:
  Transpose/1 -> A_N/L/1  "A_N/L"
  MATLAB Function1/1(A_LN) -> Transpose/1  "A_LN"
  mean motion/1 -> MATLAB Function1/2(n)
  Clock/1 -> Add/1
  Add/1 -> MATLAB Function1/1(t)
  Constant1/1 -> Add/2

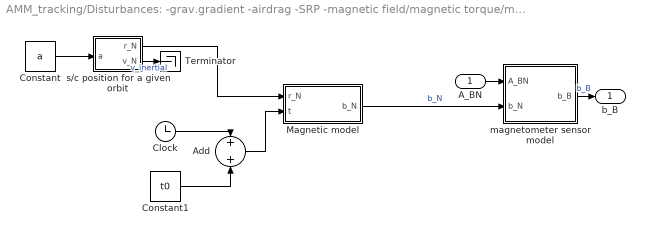
== system AMM_tracking/Disturbances: -grav.gradient -airdrag -SRP -magnetic field/magnetic torque/magnetic model ==
  A_BN : Inport
  Add : Sum
  Clock : Clock
  Constant : Constant  Value=a
  Constant1 : Constant  Value=t0
  Magnetic model : MATLAB Function  TreatAsAtomicUnit=on
  Terminator : Terminator
  magnetometer sensor model : Subsystem
  s/c position for a given orbit : Subsystem
  b_B : Outport
  wires:
  magnetometer sensor model/1(b_B) -> b_B/1  "b_B"
  Magnetic model/1(b_N) -> magnetometer sensor model/2(b_N)  "b_N"
  A_BN/1 -> magnetometer sensor model/1(A_BN)
  s/c position for a given orbit/1(r_N) -> Magnetic model/1(r_N)
  Clock/1 -> Add/1
  Constant/1 -> s/c position for a given orbit/1(a)
  s/c position for a given orbit/2(v_N) -> Terminator/1  "v_inertial"
  Constant1/1 -> Add/2
  Add/1 -> Magnetic model/2(t)

== system AMM_tracking/Sensors DCM/s//c position for a given orbit/orb_elements dynamics ==
  a : Inport
  Integrator : Integrator  InitialCondition=init_orb
  sat motion : MATLAB Function  TreatAsAtomicUnit=on
  orb_elements : Outport
  wires:
  Integrator/1 -> sat motion/2(orb_elements), orb_elements/1  "orb_elements"
  sat motion/1(orb_elements_dot) -> Integrator/1
  a/1 -> sat motion/1(a)

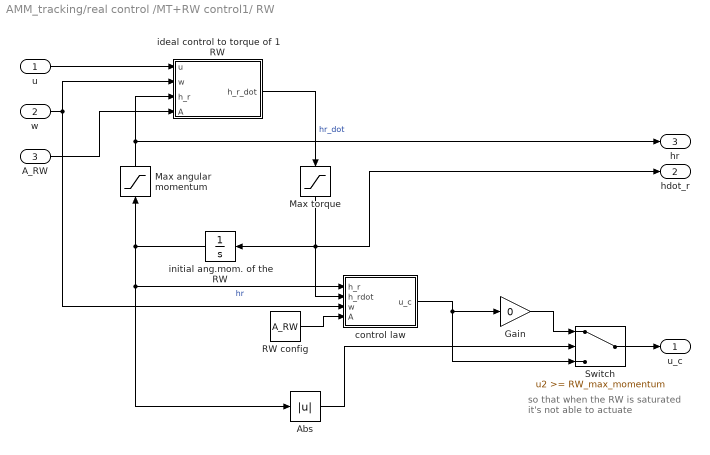
== system AMM_tracking/real control /MT+RW control1/ RW ==
  note: so that when the RW is saturated
      | it's not able to actuate
  u : Inport
  w : Inport  Port=2
  A_RW : Inport  Port=3
  Abs : Abs
  Gain : Gain  Gain=0
  Max angular momentum : Saturate  UpperLimit=RW_max_momentum  LowerLimit=-RW_max_momentum
  Max torque : Saturate  UpperLimit=RW_max_torque  LowerLimit=-RW_max_torque
  RW config : Constant  Value=A_RW
  Switch : Switch  Threshold=RW_max_momentum
  control law : MATLAB Function  TreatAsAtomicUnit=on
  ideal control to torque of 1 RW : MATLAB Function  TreatAsAtomicUnit=on
  "initial ang.mom. of the RW " : Integrator  InitialCondition=init_hr
  u_c : Outport
  hdot_r : Outport  Port=2
  hr : Outport  Port=3
  wires:
  u/1 -> ideal control to torque of 1 RW/1(u)
  w/1 -> ideal control to torque of 1 RW/2(w), control law/3(w)
  ideal control to torque of 1 RW/1(h_r_dot) -> Max torque/1  "hr_dot"
  "initial ang.mom. of the RW "/1 -> Max angular momentum/1, Abs/1, control law/1(h_r)  "hr"
  Max torque/1 -> "initial ang.mom. of the RW "/1, control law/2(h_rdot), hdot_r/1
  Max angular momentum/1 -> hr/1, ideal control to torque of 1 RW/3(h_r)
  RW config/1 -> control law/4(A)
  A_RW/1 -> ideal control to torque of 1 RW/4(A)
  Abs/1 -> Switch/2
  Switch/1 -> u_c/1
  control law/1(u_c) -> Gain/1, Switch/3
  Gain/1 -> Switch/1

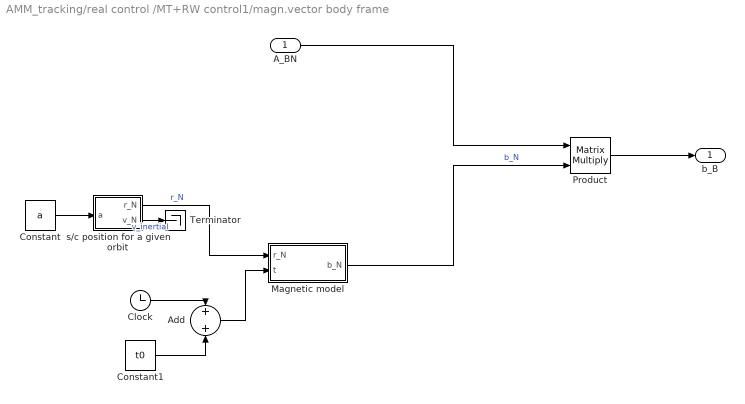
== system AMM_tracking/real control /MT+RW control1/magn.vector body frame ==
  A_BN : Inport
  Add : Sum
  Clock : Clock
  Constant : Constant  Value=a
  Constant1 : Constant  Value=t0
  Magnetic model : MATLAB Function  TreatAsAtomicUnit=on
  Product : Product  Multiplication=Matrix(*)
  Terminator : Terminator
  s/c position for a given orbit : Subsystem
  b_B : Outport
  wires:
  Magnetic model/1(b_N) -> Product/2  "b_N"
  s/c position for a given orbit/1(r_N) -> Magnetic model/1(r_N)  "r_N"
  Constant/1 -> s/c position for a given orbit/1(a)
  s/c position for a given orbit/2(v_N) -> Terminator/1  "v_inertial"
  Clock/1 -> Add/1
  Add/1 -> Magnetic model/2(t)
  Constant1/1 -> Add/2
  A_BN/1 -> Product/1
  Product/1 -> b_B/1

== system AMM_tracking/Disturbances: -grav.gradient -airdrag -SRP -magnetic field/air drag/s//c position for a given orbit/orb_elements dynamics ==
  a : Inport
  Integrator : Integrator  InitialCondition=init_orb
  sat motion : MATLAB Function  TreatAsAtomicUnit=on
  orb_elements : Outport
  wires:
  Integrator/1 -> sat motion/2(orb_elements), orb_elements/1  "orb_elements"
  sat motion/1(orb_elements_dot) -> Integrator/1
  a/1 -> sat motion/1(a)

== system AMM_tracking/Disturbances: -grav.gradient -airdrag -SRP -magnetic field/magnetic torque/magnetic model/magnetometer sensor model ==
  A_BN : Inport
  b_N : Inport  Port=2
  Product : Product  Multiplication=Matrix(*)
  b_B : Outport
  wires:
  A_BN/1 -> Product/1
  b_N/1 -> Product/2
  Product/1 -> b_B/1

== system AMM_tracking/Disturbances: -grav.gradient -airdrag -SRP -magnetic field/magnetic torque/magnetic model/s//c position for a given orbit ==
  a : Inport
  Earth's position : MATLAB Function  TreatAsAtomicUnit=on
  orb_elements dynamics : Subsystem
  r_N : Outport
  v_N : Outport  Port=2
  wires:
  Earth's position/1(r_N) -> r_N/1  "r_N"
  orb_elements dynamics/1(orb_elements) -> Earth's position/2(orb_elements)
  a/1 -> orb_elements dynamics/1(a), Earth's position/1(a)  "a"
  Earth's position/2(v_N) -> v_N/1

== system AMM_tracking/real control /MT+RW control1/magn.vector body frame/s//c position for a given orbit ==
  a : Inport
  Earth's position : MATLAB Function  TreatAsAtomicUnit=on
  orb_elements dynamics : Subsystem
  r_N : Outport
  v_N : Outport  Port=2
  wires:
  Earth's position/1(r_N) -> r_N/1  "r_N"
  orb_elements dynamics/1(orb_elements) -> Earth's position/2(orb_elements)
  a/1 -> orb_elements dynamics/1(a), Earth's position/1(a)  "a"
  Earth's position/2(v_N) -> v_N/1

== system AMM_tracking/Disturbances: -grav.gradient -airdrag -SRP -magnetic field/magnetic torque/magnetic model/s//c position for a given orbit/orb_elements dynamics ==
  a : Inport
  Integrator : Integrator  InitialCondition=init_orb
  sat motion : MATLAB Function  TreatAsAtomicUnit=on
  orb_elements : Outport
  wires:
  Integrator/1 -> sat motion/2(orb_elements), orb_elements/1  "orb_elements"
  sat motion/1(orb_elements_dot) -> Integrator/1
  a/1 -> sat motion/1(a)

== system AMM_tracking/real control /MT+RW control1/magn.vector body frame/s//c position for a given orbit/orb_elements dynamics ==
  a : Inport
  Integrator : Integrator  InitialCondition=init_orb
  sat motion : MATLAB Function  TreatAsAtomicUnit=on
  orb_elements : Outport
  wires:
  Integrator/1 -> sat motion/2(orb_elements), orb_elements/1  "orb_elements"
  sat motion/1(orb_elements_dot) -> Integrator/1
  a/1 -> sat motion/1(a)

== matlab function AMM_tracking/real control /MT+RW control1/ RW/control law ==
  data: h_r input; h_rdot input; w input; u_c output; A input
function u_c = fcn(h_r,h_rdot,w,A)

u_c = zeros(3,1);
u_c = -A*h_rdot-cross(w,A*h_r);

== matlab function AMM_tracking/Gyro Model/Gyro model Input angular velocity of the spacecraft with output the gyro torque/MATLAB Function1 ==
  data: x input; om input; x_dot output; M output
function [x_dot,M]  = Gyro(x,om)
%gyro inertia parameters 
Ir = 1e-7; 
Iz = 2e-7;
%tuning parameter for visco-elastic reaction torque
k_gyro=10;
%tuning law for c for fastest convergence
c_gyro = 2*sqrt(k_gyro*Iz); 
om_x = om(1); 
om_y = om(2); 
om_z = om(3); 
%angular velocity of gyro wheel
om_r = 100*pi/180;

% defining the theta_i and \dot theta_i 
x_dot = zeros(6,1); 

th_x = x(1); 
th_y = x(2); 
th_z = x(3);
va_x = x(4);
va_y = x(5); 
va_z = x(6); 
%3 gyro dynamics expressed as 1st order differential equation
x_dot(1) = va_x;
x_dot(2) = va_y; 
x_dot(3) = va_z;
x_dot(4) = -(c_gyro/Iz)*va_x-(k_gyro/Iz)*th_x-(Ir/Iz)*om_r*om_x;
x_dot(5) = -(c_gyro/Iz)*va_y-(k_gyro/Iz)*th_y-(Ir/Iz)*om_r*om_y;
x_dot(6) = -(c_gyro/Iz)*va_z-(k_gyro/Iz)*th_z-(Ir/Iz)*om_r*om_z;
%gyro outputs 
x_dot=[x_dot(1) x_dot(2) x_dot(3) x_dot(4) x_dot(5) x_dot(6)]';
%feedback torque applied to the gyros 
M_x = -k_gyro*th_x-c_gyro*va_x;
M_y = -k_gyro*th_y-c_gyro*va_y;
M_z = -k_gyro*th_z-c_gyro*va_z;

M = [M_x M_y M_z]'; 


end

== matlab function AMM_tracking/Gyro Model/Low Pass Filter for the measured angular velocity ==
  data: w_est input; w_meas input; u input; west_dot output; alpha input
function west_dot = dynamics(w_est,w_meas,u,alpha)

J1 = 0.1054;
J2 = 0.0914;
J3 = 0.0541;

west_dot = zeros(size(w_est));

west_dot(1) =       (J2 - J3)/J1 * w_est(2) * w_est(3) + u(1)/J1 - ...
                alpha*(w_est(1)-w_meas(1))/J1;
west_dot(2) =       (J3 - J1)/J2 * w_est(1) * w_est(3) + u(2)/J2 - ...
                alpha*(w_est(2)-w_meas(2))/J2;
west_dot(3) =       (J1 - J2)/J3 * w_est(1) * w_est(2) + u(3)/J3 - ...
                alpha*(w_est(3)-w_meas(3))/J3;

== matlab function AMM_tracking/Sensors DCM/Earth Horizon ==
  data: A_BN input; hB output; r input; hN output; dtheta input; dir input
function [hB, hN] = EH_sensor(A_BN, r, dtheta, dir)    
    
    hN = -r/norm(r);
    
    % Matrix error
    dir = dir/norm(dir);
    
        e_hat       = zeros (3);

        e_hat (1,2) = - dir(3);
        e_hat (1,3) =   dir(2);
        e_hat (2,1) =   dir(3);
        e_hat (2,3) = - dir(1);
        e_hat (3,1) = - dir(2);
        e_hat (3,2) =   dir(1);
    
    A_err = eye(3) - sin(dtheta)*e_hat + (1-cos(dtheta))* e_hat*e_hat; 
    
%     A_err = [        cos(err)^2, cos(err)*sin(err)^2 + sin(err)*cos(err),       -cos(err)^2*sin(err) + sin(err)^2; ...
%              -sin(err)*cos(err),                -sin(err)^3 + cos(err)^2, sin(err)^2*cos(err) + cos(err)*sin(err); ...
%                        sin(err),                      -cos(err)*sin(err),                            cos(err)^2 ];
    
    hB = A_err * A_BN * hN;

end

== matlab function AMM_tracking/Sensors DCM/Magneto Sensor ==
  data: A_BN input; bB output; r input; noise input; bN output; dtheta input; dir input; t input
function [bB, bN] = Magn_sensor(A_BN, r, noise, dtheta, dir, t)    
    
    H0    = sqrt( (-29615)^2 + (-1728)^2 + (5186)^2 ) * 1E-9;
    R     = 6371200;                            % Earth radious   [m]
    omega = (2*pi)/(23*3600+56*60+4);           % Angular velocitiy Earth [rad/s]    
    
    r_vN  = r/norm(r);
        
    m_v   = [ sin(11.5*pi/180)*cos(omega*t); ...
              sin(11.5*pi/180)*sin(omega*t); ...
              cos(11.5*pi/180) ];
    
    bN    = (R^3 * H0 / norm(r)^3) * (3* (dot(m_v, r_vN) * r_vN) - m_v);
    
    % Matrix error
    dir = dir/norm(dir);
    
        e_hat       = zeros (3);

        e_hat (1,2) = - dir(3);
        e_hat (1,3) =   dir(2);
        e_hat (2,1) =   dir(3);
        e_hat (2,3) = - dir(1);
        e_hat (3,1) = - dir(2);
        e_hat (3,2) =   dir(1);
    
    A_err = eye(3) - sin(dtheta)*e_hat + (1-cos(dtheta))* e_hat*e_hat; 
   
%     A_err = [        cos(err)^2, cos(err)*sin(err)^2 + sin(err)*cos(err),       -cos(err)^2*sin(err) + sin(err)^2; ...
%              -sin(err)*cos(err),                -sin(err)^3 + cos(err)^2, sin(err)^2*cos(err) + cos(err)*sin(err); ...
%                        sin(err),                      -cos(err)*sin(err),                            cos(err)^2 ];
      
    bB   = A_err * A_BN * bN + noise;
    bB = bB/norm(bB);
    bN = bN/norm(bN);

end

== matlab function AMM_tracking/Sensors DCM/s//c position for a given orbit/Earth's position ==
  data: a input; orb_elements input; r_N output; v_N output
function [r_N,v_N]  = Earth_pos(a,orb_elements)

mu = 3.986004418e14;

e_mod = orb_elements(1);
i     = orb_elements(2);
Omega = orb_elements(3);
omega = orb_elements(4);
theta = orb_elements(5);


h_mod = sqrt(mu*a*(1-e_mod^2));
    
e_unit = rotation_matrix_R3(-Omega) * ...
         rotation_matrix_R1(-i) * ...
         rotation_matrix_R3(-omega) * [1;0;0];
p_unit = rotation_matrix_R3(-Omega) * ...
         rotation_matrix_R1(-i) * ...
         rotation_matrix_R3(-omega) * [0;1;0];
     
r_mod_0 = h_mod^2/mu/(1+e_mod*cos(theta));
r_N       = r_mod_0 * ( cos(theta) * e_unit  +  sin(theta) * p_unit );
v_r     = mu/h_mod * e_mod*sin(theta);
v_theta = mu/h_mod * (1 + e_mod*cos(theta));
v_N       = v_r     * (  cos(theta) * e_unit  +  sin(theta) * p_unit )+ ...
          v_theta * ( -sin(theta) * e_unit  +  cos(theta) * p_unit );
end


function R1 = rotation_matrix_R1(alpha)
%{
rotation_matrix_R1: computes rotation matrix of angle alpha around x axis

INPUT:
	alpha[1]                Angle rotated
                                [rad]

OUTPUT:
    R1 [3x3]                Rotation matrix
                                [(3x3) x -]
%}

R1 = zeros(3);

R1(1,1) = 1;
R1(2,2) =  cos(alpha);
R1(2,3) =  sin(alpha);
R1(3,2) = -sin(alpha);
R1(3,3) =  cos(alpha);
end


function R3 = rotation_matrix_R3(alpha)
%{
rotation_matrix_R3: computes rotation matrix of angle alpha around z axis

INPUT:
	alpha[1]                Angle rotated
                                [rad]

OUTPUT:
    R3 [3x3]                Rotation matrix
                                [(3x3) x -]

%}

R3 = zeros(3);

R3(1,1) =  cos(alpha);
R3(1,2) =  sin(alpha);
R3(2,1) = -sin(alpha);
R3(2,2) =  cos(alpha);
R3(3,3) =  1;
end

== matlab function AMM_tracking/real control /MT+RW control1/ RW/ideal control to torque of 1 RW ==
  data: u input; h_r_dot output; w input; h_r input; A input
function h_r_dot = fcn(u,w,h_r,A)

Apseudo_inv = pinv(A);

h_r_dot = 0;
h_r_dot = -Apseudo_inv*(u+cross(w,A*h_r));

== matlab function AMM_tracking/Disturbances: -grav.gradient -airdrag -SRP -magnetic field/SRP moment/Sun direction wrt s//c body frame/Sun's direction ==
  data: t input; S_N output
function S_N = fcn(t)

%% data
Rs = 149597870700; %[m] but we can substitute it by 1 so we have a unitary vector
Rs = 1;
epsilon = 23.45 * pi/180; %[rad]
T = 365.25*24*3600; %[s]
nsun = 2*pi/T; % [s^-1]

%% 
S_N = Rs * [cos(nsun*t);
            sin(nsun*t)*cos(epsilon);
            sin(nsun*t)*sin(epsilon);];

end

== matlab function AMM_tracking/real control /MT+RW control1/ideal control law ==
  data: M input; b input; m output
function m = fcn(M,b)

B = [0, -1, 0;
    1, 0, 0;
    b(1), b(2), b(3)
    ];


m = 1/b(3)*B*M;

end

== matlab function AMM_tracking/real control /MT+RW control1/magn.vector body frame/Magnetic model ==
  data: r_N input; b_N output; t input
function b_N = fcn(r_N,t)
% coefficients
IGRF = '2000';
switch IGRF
    case '1995'
        g0_1 = -29682e-9;
        g1_1 = -1789e-9;
        h1_1 = 5318e-9;
    case '2000'
        g0_1 = -29615e-9;
        g1_1 = -1728e-9;
        h1_1 = 5186e-9;
end


w = 360/(24*3600) * pi/180; %[rad/s] angular rotation speed of Earth
decl = 11.5*pi/180; %[rad]
R = 6371.2e3; %equatorial radius [m]
r = norm(r_N);
rr_unit = r_N/r; %unitary vector

H0 = sqrt(g0_1^2 + g1_1^2 + h1_1^2);
m = [
    sin(decl)*cos(w*t);
    sin(decl)*sin(w*t);
    cos(decl)
    ]; %unit vector along dipole axis

b_N = R^3*H0/r^3*(3*(dot(m,rr_unit))*rr_unit - m); %Earth's MF in the inertial frame

== matlab function AMM_tracking/real control /MT+RW control1/magn.vector body frame/s//c position for a given orbit/Earth's position ==
  data: a input; orb_elements input; r_N output; v_N output
function [r_N,v_N]  = Earth_pos(a,orb_elements)

mu = 3.986004418e14;

e_mod = orb_elements(1);
i     = orb_elements(2);
Omega = orb_elements(3);
omega = orb_elements(4);
theta = orb_elements(5);


h_mod = sqrt(mu*a*(1-e_mod^2));
    
e_unit = rotation_matrix_R3(-Omega) * ...
         rotation_matrix_R1(-i) * ...
         rotation_matrix_R3(-omega) * [1;0;0];
p_unit = rotation_matrix_R3(-Omega) * ...
         rotation_matrix_R1(-i) * ...
         rotation_matrix_R3(-omega) * [0;1;0];
     
r_mod_0 = h_mod^2/mu/(1+e_mod*cos(theta));
r_N       = r_mod_0 * ( cos(theta) * e_unit  +  sin(theta) * p_unit );
v_r     = mu/h_mod * e_mod*sin(theta);
v_theta = mu/h_mod * (1 + e_mod*cos(theta));
v_N       = v_r     * (  cos(theta) * e_unit  +  sin(theta) * p_unit )+ ...
          v_theta * ( -sin(theta) * e_unit  +  cos(theta) * p_unit );
end


function R1 = rotation_matrix_R1(alpha)
%{
rotation_matrix_R1: computes rotation matrix of angle alpha around x axis

INPUT:
	alpha[1]                Angle rotated
                                [rad]

OUTPUT:
    R1 [3x3]                Rotation matrix
                                [(3x3) x -]
%}

R1 = zeros(3);

R1(1,1) = 1;
R1(2,2) =  cos(alpha);
R1(2,3) =  sin(alpha);
R1(3,2) = -sin(alpha);
R1(3,3) =  cos(alpha);
end


function R3 = rotation_matrix_R3(alpha)
%{
rotation_matrix_R3: computes rotation matrix of angle alpha around z axis

INPUT:
	alpha[1]                Angle rotated
                                [rad]

OUTPUT:
    R3 [3x3]                Rotation matrix
                                [(3x3) x -]

%}

R3 = zeros(3);

R3(1,1) =  cos(alpha);
R3(1,2) =  sin(alpha);
R3(2,1) = -sin(alpha);
R3(2,2) =  cos(alpha);
R3(3,3) =  1;
end

== matlab function AMM_tracking/real control /MT+RW control1/magn.vector body frame/s//c position for a given orbit/orb_elements dynamics/sat motion ==
  data: a input; orb_elements input; orb_elements_dot output
function orb_elements_dot = orbit(a,orb_elements)

mu = 3.986004418e14;

e     = orb_elements(1);
i     = orb_elements(2);
O = orb_elements(3);
o = orb_elements(4);
theta = orb_elements(5); %true anomaly


n     = sqrt( mu / a^3 ); %mean motion: angular speed required to complete 1 orbit

orb_elements_dot    = zeros (size(orb_elements));

orb_elements_dot(5) = n * (1 + e*cos(theta))^2 / (1 - e^2)^(3/2);

== matlab function AMM_tracking/Disturbances: -grav.gradient -airdrag -SRP -magnetic field/gravity gradient/A_N//L/MATLAB Function1 ==
  data: t input; A_LN output; n input
function A_LN = fcn(t,n)

% mu = 3.986004418e14;
% n = sqrt( mu / a^3 ); %is this the nº of revolutions per orbit?
A_LN = [cos(n*t) sin(n*t) 0;
    -sin(n*t) cos(n*t) 0;
    0 0 1;
    ];

== matlab function AMM_tracking/Sun direction wrt s//c body frame2/Sun's direction ==
  data: t input; S_N output
function S_N = fcn(t)

%% data
Rs = 149597870700; %[m] but we can substitute it by 1 so we have a unitary vector
% Rs = 1;
epsilon = 23.45 * pi/180; %[rad]
T = 365.25*24*3600; %[s]
nsun = 2*pi/T; % [s^-1]

%% 
s_N = Rs * [cos(nsun*t);
            sin(nsun*t)*cos(epsilon);
            sin(nsun*t)*sin(epsilon)];
S_N = s_N/norm(s_N);

end

== matlab function AMM_tracking/reference DCM2/DCM_ref ==
  data: v_ref input; A_d output; r_sc input
function A_d = DCM_ref (v_ref, r_sc)

% r_sc = r_sc/norm(r_sc);
 
v1 = v_ref/norm(v_ref); 
v3 = cross(v1,r_sc)/norm(cross(v1,r_sc));
v2 = cross(v3,v1);

% A_d = [v1'; v2'; v3'];
A_d = [v1, v2, v3];

end

== matlab function AMM_tracking/DCM feedback control2/DCM feedback ==
  data: w input; A_e input; K1 input; K2 input; u output; J input
function u = DCM_fbk_control(w,A_e,K1,K2,J)

mu_sun = 1.32712440018e20;
a_sun = 149.6e9;

w_ref = [0; 0; -sqrt(mu_sun/a_sun^3) ];
I_x = J(1);
I_y = J(2);
I_z = J(3);

% u = -K1*w - K2*[A_e(2,3)-A_e(3,2); A_e(3,1)-A_e(1,3); A_e(1,2)-A_e(2,1)];
u = - K1 * [I_x;I_y;I_z].*(w - w_ref) ...
    - K2 * [I_x;I_y;I_z].*[A_e(2,3)-A_e(3,2); A_e(3,1)-A_e(1,3); A_e(1,2)-A_e(2,1)] ...
    + cross ( w, [I_x;I_y;I_z].*w );
%     - K3 * sign(w) ...
%     + K2 * ( (trace(A_e)-1)*[A_e(3,2)-A_e(2,3); A_e(1,3)-A_e(3,1); A_e(2,1)-A_e(1,2)] - w ) ...

% Avoid excesive rotational rate problematic for attitude acquisition (0.5 deg/s)
u_sat_max = - K1 * [I_x;I_y;I_z].*(w - 0.45*pi/180*[1;1;1]/sqrt(3)) ...
            + cross ( w, [I_x;I_y;I_z].*w );
u_sat_min = - K1 * [I_x;I_y;I_z].*(w + 0.45*pi/180*[1;1;1]/sqrt(3)) ...
            + cross ( w, [I_x;I_y;I_z].*w );
for i = 1:3
    if ( u(i)*w(i) > 0 ) && ( abs(w(i)) > 0.4*pi/180/sqrt(3) )
%         u(i) = - K1*w(i);
%         u(i) = - K1*sign(w(i))*(abs(w(i)) - 0.45*pi/180);
        if w(i)>0
            u(i) = u_sat_max(i);
        else
            u(i) = u_sat_min(i);
        end
    end
end
end

== matlab function AMM_tracking/Disturbances: -grav.gradient -airdrag -SRP -magnetic field/magnetic torque/magnetic model/Magnetic model ==
  data: r_N input; b_N output; t input
function b_N = fcn(r_N,t)
% coefficients
IGRF = '2000';
switch IGRF
    case '1995'
        g0_1 = -29682e-9;
        g1_1 = -1789e-9;
        h1_1 = 5318e-9;
    case '2000'
        g0_1 = -29615e-9;
        g1_1 = -1728e-9;
        h1_1 = 5186e-9;
end


w = 360/(24*3600) * pi/180; %[rad/s] angular rotation speed of Earth
decl = 11.5*pi/180; %[rad]
R = 6371.2e3; %equatorial radius [m]
r = norm(r_N);
rr_unit = r_N/r; %unitary vector

H0 = sqrt(g0_1^2 + g1_1^2 + h1_1^2);
m = [
    sin(decl)*cos(w*t);
    sin(decl)*sin(w*t);
    cos(decl)
    ]; %unit vector along dipole axis

b_N = R^3*H0/r^3*(3*(dot(m,rr_unit))*rr_unit - m); %Earth's MF in the inertial frame

== matlab function AMM_tracking/Disturbances: -grav.gradient -airdrag -SRP -magnetic field/gravity gradient/gravity gradient ==
  data: A_BL input; G output; J input; n input
function G = fcn(A_BL,J,n)

%Data
% mu = 3.986004418e14;
% n  = sqrt(mu/a^3);
% %Moment of inertia of s/c
% Ix = 100.9e-2; %[kg m^2]
% Iy = 25.1e-2;
% Iz = 91.6e-2; 
Ix = J(1);
Iy = J(2);
Iz = J(3);
c = A_BL * [1;0;0];

G = zeros(3,1);
G(1) = 3*n^2 * (Iz - Iy)*c(3)*c(2);
G(2) = 3*n^2 * (Ix - Iz)*c(1)*c(3);
G(3) = 3*n^2 * (Iy - Ix)*c(2)*c(1);

end
